simulink model "NN_SMC_Position"  (R2024b)
settings: Solver=ode4  StartTime=0.0  StopTime=200  FixedStep=0.01  RelTol=1e-3
InitFcn:
  |             % distance between camera and world frame
  | ang_initial = [0.0 0.0 0.0];  % initial orientation, [pi 0 pi/2]
  | 
  | init_pose = [C ; ang_initial'];
  | 
  | dT=0.25;
  | g = 9.81;
  | mass = 1; L = 0.2;
  | Ix = 0.008;
  | Iy = 0.008;
  | Iz = 0.017;
  | c = 0.088;
undefined symbols (not defined in the file): C
libraries: ros2lib x2
settings Model: Creator=k513  LastModifiedBy=mohsen
settings DataIOCC: ReturnWorkspaceOutputs=off
settings ModelReferenceCC: EnableRefExpFcnMdlSchedulingChecks=on
settings RTWCC: GPUComputeCapability=3.5

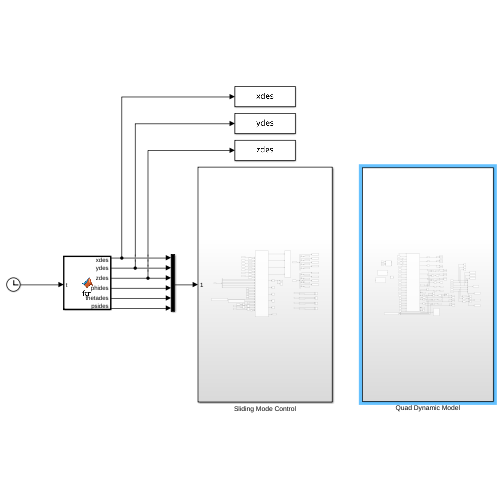
[thumbnail: Simulink's stored preview of the top-level diagram]
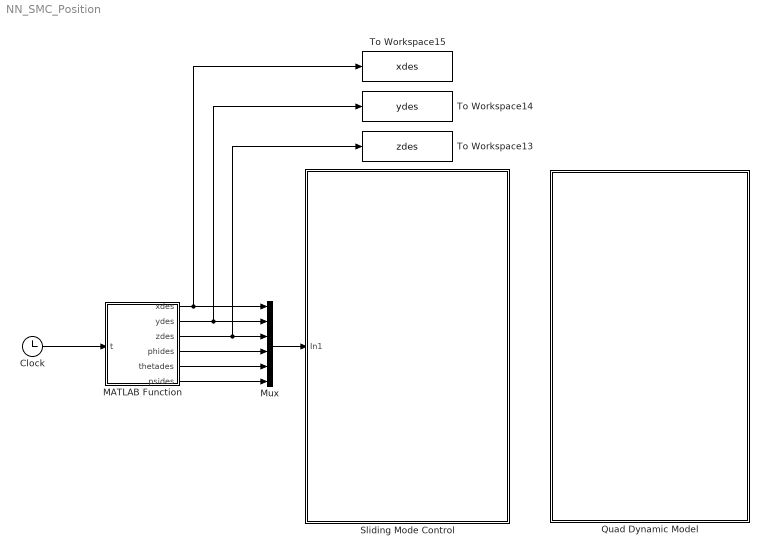
== system NN_SMC_Position ==
  Clock : Clock
  MATLAB Function : MATLAB Function  TreatAsAtomicUnit=on
  Mux : Mux  Inputs=6
  Quad Dynamic Model : Subsystem
  Sliding Mode Control : Subsystem
  To Workspace13 : ToWorkspace  VariableName=zdes  SampleTime=-1
      settings: Save2DSignal=2-D array (concatenate along first dimension)
  To Workspace14 : ToWorkspace  VariableName=ydes  SampleTime=-1
      settings: Save2DSignal=2-D array (concatenate along first dimension)
  To Workspace15 : ToWorkspace  VariableName=xdes  SampleTime=-1
      settings: Save2DSignal=2-D array (concatenate along first dimension)
  wires:
  Clock/1 -> MATLAB Function/1(t)
  Mux/1 -> Sliding Mode Control/1(In1)
  MATLAB Function/1(xdes) -> Mux/1, To Workspace15/1
  MATLAB Function/2(ydes) -> Mux/2, To Workspace14/1
  MATLAB Function/3(zdes) -> Mux/3, To Workspace13/1
  MATLAB Function/4(phides) -> Mux/4
  MATLAB Function/5(thetades) -> Mux/5
  MATLAB Function/6(psides) -> Mux/6

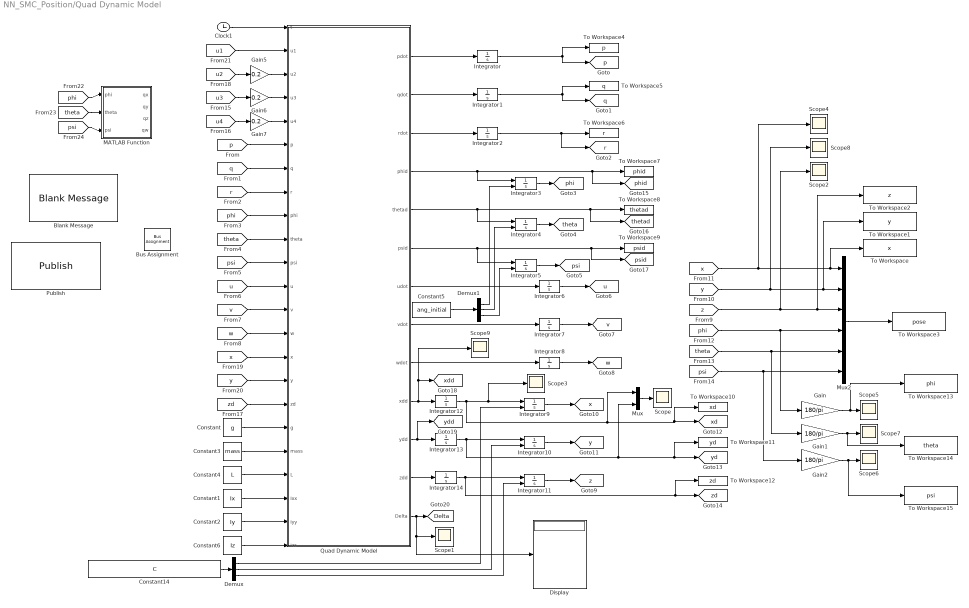
== system NN_SMC_Position/Quad Dynamic Model ==
  Blank Message : ros2lib/Blank Message  messageClass=Message  entityType=geometry_msgs/PoseStamped  messageType=geometry_msgs/PoseStamped  SampleTime=inf
  Bus Assignment : BusAssignment  AssignedSignals=signal1
  Clock1 : Clock
  Constant : Constant  Value=g
  Constant1 : Constant  Value=Ix
  Constant14 : Constant  Value=C
  Constant2 : Constant  Value=Iy
  Constant3 : Constant  Value=mass
  Constant4 : Constant  Value=L
  Constant5 : Constant  Value=ang_initial
  Constant6 : Constant  Value=Iz
  Demux : Demux  Outputs=3
  Demux1 : Demux  Outputs=3
  Display : Display
  Gain : Gain  Gain=180/pi
  Gain1 : Gain  Gain=180/pi
  Gain2 : Gain  Gain=180/pi
  Gain5 : Gain  Gain=0.2
  Gain6 : Gain  Gain=0.2
  Gain7 : Gain  Gain=0.2
  Integrator : Integrator  InitialCondition=-0.003775510005653
  Integrator1 : Integrator  InitialCondition=0.003931066952646
  Integrator{3..5,9..11} (6 alike) : Integrator  InitialConditionSource=external
  Integrator{6..8,12..14} (6 alike) : Integrator
  Integrator2 : Integrator  InitialCondition=0.005723309703171
  MATLAB Function : MATLAB Function  TreatAsAtomicUnit=on
  Mux : Mux  Inputs=2
  Mux2 : Mux  Inputs=6
  Publish : ros2lib/Publish  topicSource=Select from ROS network  topic=/my_topic  messageType=geometry_msgs/Point  QOSHistory=Keep last  QOSDepth=1  QOSReliability=Reliable  QOSDurability=Volatile  QOSDeadline=Inf  QOSLifespan=Inf  QOSLiveliness=Automatic  QOSLeaseDuration=Inf  QOSAvoidROSNamespaceConventions=off
  Quad Dynamic Model : MATLAB Function  TreatAsAtomicUnit=on
  Scope{,1..9} (10 alike) : Scope
  To Workspace : ToWorkspace  VariableName=x  SampleTime=-1
      settings: Save2DSignal=2-D array (concatenate along first dimension)
  To Workspace1 : ToWorkspace  VariableName=y  SampleTime=-1
      settings: Save2DSignal=2-D array (concatenate along first dimension)
  To Workspace10 : ToWorkspace  VariableName=xd  SampleTime=-1
  To Workspace11 : ToWorkspace  VariableName=yd  SampleTime=-1
  To Workspace12 : ToWorkspace  VariableName=zd  SampleTime=-1
  To Workspace13 : ToWorkspace  VariableName=phi  SampleTime=-1
      settings: Save2DSignal=2-D array (concatenate along first dimension)
  To Workspace14 : ToWorkspace  VariableName=theta  SampleTime=-1
      settings: Save2DSignal=2-D array (concatenate along first dimension)
  To Workspace15 : ToWorkspace  VariableName=psi  SampleTime=-1
      settings: Save2DSignal=2-D array (concatenate along first dimension)
  To Workspace2 : ToWorkspace  VariableName=z  SampleTime=-1
      settings: Save2DSignal=2-D array (concatenate along first dimension)
  To Workspace3 : ToWorkspace  VariableName=pose  SampleTime=-1
      settings: Save2DSignal=2-D array (concatenate along first dimension)
  To Workspace4 : ToWorkspace  VariableName=p  SampleTime=-1
  To Workspace5 : ToWorkspace  VariableName=q  SampleTime=-1
  To Workspace6 : ToWorkspace  VariableName=r  SampleTime=-1
  To Workspace7 : ToWorkspace  VariableName=phid  SampleTime=-1
  To Workspace8 : ToWorkspace  VariableName=thetad  SampleTime=-1
  To Workspace9 : ToWorkspace  VariableName=psid  SampleTime=-1
  tag scope: Delta=global, p=global, phi=global, phid=global, psi=global, psid=global, q=global, r=global, theta=global, thetad=global, u=global, v=global, w=global, x=global, xd=global, xdd=global, y=global, yd=global, ydd=global, z=global, zd=global
  wires:
  Quad Dynamic Model/1(pdot) -> Integrator/1
  Quad Dynamic Model/2(qdot) -> Integrator1/1
  Quad Dynamic Model/3(rdot) -> Integrator2/1
  Quad Dynamic Model/4(phid) -> Integrator3/1, [phid], To Workspace7/1
  Quad Dynamic Model/5(thetad) -> Integrator4/1, [thetad], To Workspace8/1
  Quad Dynamic Model/7(udot) -> Integrator6/1
  Quad Dynamic Model/9(wdot) -> Integrator8/1
  Quad Dynamic Model/10(xdd) -> Integrator12/1, Scope9/1, [xdd]
  Quad Dynamic Model/11(ydd) -> Integrator13/1, [ydd]
  Quad Dynamic Model/12(zdd) -> Integrator14/1
  Integrator1/1 -> To Workspace5/1, [q]
  Integrator2/1 -> To Workspace6/1, [r]
  Integrator3/1 -> [phi]
  Integrator4/1 -> [theta]
  Integrator5/1 -> [psi]
  Integrator6/1 -> [u]
  Integrator7/1 -> [v]
  Integrator8/1 -> [w]
  [p] -> Quad Dynamic Model/6(p)
  [q] -> Quad Dynamic Model/7(q)
  [r] -> Quad Dynamic Model/8(r)
  [phi] -> Quad Dynamic Model/9(phi)
  [theta] -> Quad Dynamic Model/10(theta)
  [psi] -> Quad Dynamic Model/11(psi)
  [u] -> Quad Dynamic Model/12(u)
  [v] -> Quad Dynamic Model/13(v)
  [w] -> Quad Dynamic Model/14(w)
  Integrator9/1 -> [x]
  Integrator10/1 -> [y]
  Integrator11/1 -> [z]
  [u2] -> Gain5/1
  [u3] -> Gain6/1
  [u4] -> Gain7/1
  Integrator12/1 -> [xd], To Workspace10/1, Mux/1, Scope3/1, Integrator9/1
  Integrator13/1 -> [yd], To Workspace11/1, Mux/2, Integrator10/1
  Integrator14/1 -> [zd], To Workspace12/1, Integrator11/1
  Quad Dynamic Model/6(psid) -> To Workspace9/1, [psid], Integrator5/1
  Demux/1 -> Integrator9/2
  Demux/2 -> Integrator10/2
  Demux/3 -> Integrator11/2
  Mux/1 -> Scope/1
  Constant14/1 -> Demux/1
  Quad Dynamic Model/8(vdot) -> Integrator7/1
  [x] -> Mux2/1, To Workspace/1, Scope4/1
  [phi] -> Gain/1, Mux2/4
  [psi] -> Mux2/6, Gain2/1
  [theta] -> Gain1/1, Mux2/5
  Gain/1 -> To Workspace13/1, Scope5/1
  Gain1/1 -> Scope7/1, To Workspace14/1
  Gain2/1 -> Scope6/1, To Workspace15/1
  [y] -> Mux2/2, To Workspace1/1, Scope8/1
  [z] -> To Workspace2/1, Mux2/3, Scope2/1
  Mux2/1 -> To Workspace3/1
  Constant/1 -> Quad Dynamic Model/18(g)
  Constant2/1 -> Quad Dynamic Model/22(Iyy)
  Constant1/1 -> Quad Dynamic Model/21(Ixx)
  Constant3/1 -> Quad Dynamic Model/19(mass)
  Constant4/1 -> Quad Dynamic Model/20(L)
  Constant5/1 -> Demux1/1
  Demux1/1 -> Integrator3/2
  Demux1/2 -> Integrator4/2
  Demux1/3 -> Integrator5/2
  Constant6/1 -> Quad Dynamic Model/23(Izz)
  Integrator/1 -> To Workspace4/1, [p]
  [u1] -> Quad Dynamic Model/2(u1)
  Gain5/1 -> Quad Dynamic Model/3(u2)
  Gain6/1 -> Quad Dynamic Model/4(u3)
  Gain7/1 -> Quad Dynamic Model/5(u4)
  [zd] -> Quad Dynamic Model/17(zd)
  Clock1/1 -> Quad Dynamic Model/1(t)
  [x] -> Quad Dynamic Model/15(x)
  [y] -> Quad Dynamic Model/16(y)
  Quad Dynamic Model/13(Delta) -> Display/1, Scope1/1, [Delta]
  [phi] -> MATLAB Function/1(phi)
  [theta] -> MATLAB Function/2(theta)
  [psi] -> MATLAB Function/3(psi)

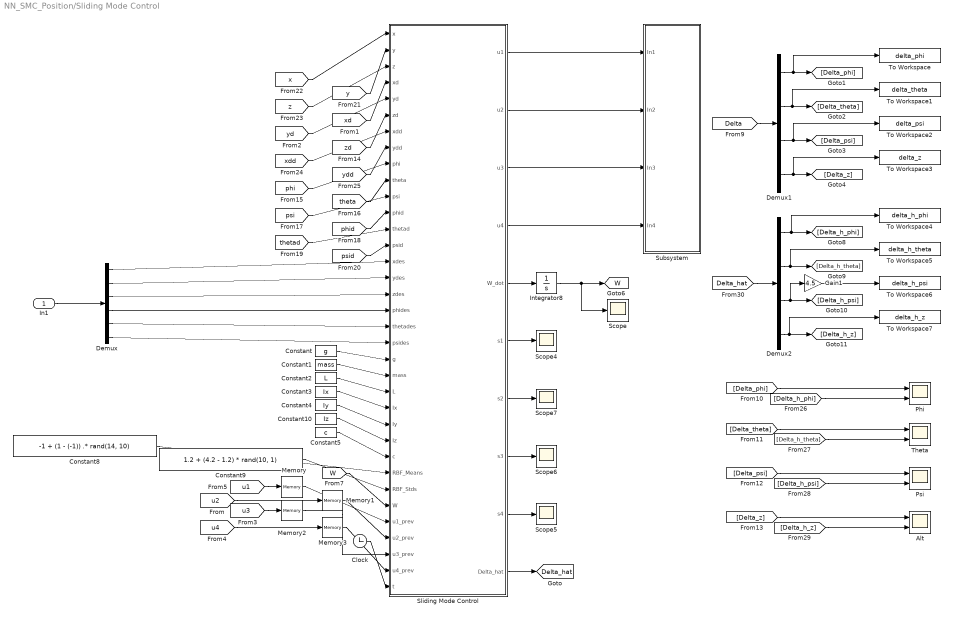
== system NN_SMC_Position/Sliding Mode Control ==
  In1 : Inport
  Alt : Scope  NumInputPorts=2
  Clock : Clock
  Constant : Constant  Value=g
  Constant1 : Constant  Value=mass
  Constant10 : Constant  Value=Iz
  Constant2 : Constant  Value=L
  Constant3 : Constant  Value=Ix
  Constant4 : Constant  Value=Iy
  Constant5 : Constant  Value=c
  Constant8 : Constant  Value=-1 + (1 - (-1)) .* rand(14, 10)
  Constant9 : Constant  Value=1.2 + (4.2 - 1.2) * rand(10, 1)
  Demux : Demux  Outputs=6
  Demux1 : Demux
  Demux2 : Demux
  Gain1 : Gain  Gain=4.5
  Integrator8 : Integrator  InitialCondition=zeros(10, 4)
  Memory{,1..3} (4 alike) : Memory
  Phi : Scope  NumInputPorts=2
  Psi : Scope  NumInputPorts=2
  Scope{,4..7} (5 alike) : Scope
  Sliding Mode Control : MATLAB Function  TreatAsAtomicUnit=on
  Subsystem : Subsystem
  Theta : Scope  NumInputPorts=2
  To Workspace : ToWorkspace  VariableName=delta_phi  SampleTime=-1
      settings: Save2DSignal=2-D array (concatenate along first dimension)
  To Workspace1 : ToWorkspace  VariableName=delta_theta  SampleTime=-1
      settings: Save2DSignal=2-D array (concatenate along first dimension)
  To Workspace2 : ToWorkspace  VariableName=delta_psi  SampleTime=-1
      settings: Save2DSignal=2-D array (concatenate along first dimension)
  To Workspace3 : ToWorkspace  VariableName=delta_z  SampleTime=-1
      settings: Save2DSignal=2-D array (concatenate along first dimension)
  To Workspace4 : ToWorkspace  VariableName=delta_h_phi  SampleTime=-1
      settings: Save2DSignal=2-D array (concatenate along first dimension)
  To Workspace5 : ToWorkspace  VariableName=delta_h_theta  SampleTime=-1
      settings: Save2DSignal=2-D array (concatenate along first dimension)
  To Workspace6 : ToWorkspace  VariableName=delta_h_psi  SampleTime=-1
      settings: Save2DSignal=2-D array (concatenate along first dimension)
  To Workspace7 : ToWorkspace  VariableName=delta_h_z  SampleTime=-1
      settings: Save2DSignal=2-D array (concatenate along first dimension)
  tag scope: Delta_hat=global, W=global
  wires:
  [theta] -> Sliding Mode Control/10(theta)
  [zd] -> Sliding Mode Control/6(zd)
  [yd] -> Sliding Mode Control/5(yd)
  [xdd] -> Sliding Mode Control/7(xdd)
  [thetad] -> Sliding Mode Control/13(thetad)
  [phid] -> Sliding Mode Control/12(phid)
  [psi] -> Sliding Mode Control/11(psi)
  [ydd] -> Sliding Mode Control/8(ydd)
  [y] -> Sliding Mode Control/2(y)
  [phi] -> Sliding Mode Control/9(phi)
  [xd] -> Sliding Mode Control/4(xd)
  [psid] -> Sliding Mode Control/14(psid)
  [x] -> Sliding Mode Control/1(x)
  [z] -> Sliding Mode Control/3(z)
  In1/1 -> Demux/1
  Demux/1 -> Sliding Mode Control/15(xdes)
  Demux/2 -> Sliding Mode Control/16(ydes)
  Demux/3 -> Sliding Mode Control/17(zdes)
  Constant/1 -> Sliding Mode Control/21(g)
  Constant1/1 -> Sliding Mode Control/22(mass)
  Constant2/1 -> Sliding Mode Control/23(L)
  Constant3/1 -> Sliding Mode Control/24(Ix)
  Constant4/1 -> Sliding Mode Control/25(Iy)
  Constant5/1 -> Sliding Mode Control/27(c)
  Demux/5 -> Sliding Mode Control/19(thetades)
  Demux/6 -> Sliding Mode Control/20(psides)
  Demux/4 -> Sliding Mode Control/18(phides)
  Constant10/1 -> Sliding Mode Control/26(Iz)
  Constant9/1 -> Sliding Mode Control/29(RBF_Stds)
  Constant8/1 -> Sliding Mode Control/28(RBF_Means)
  Sliding Mode Control/5(W_dot) -> Integrator8/1
  [u1] -> Memory/1
  [u2] -> Memory1/1
  [u3] -> Memory2/1
  [u4] -> Memory3/1
  Sliding Mode Control/6(s1) -> Scope4/1
  Sliding Mode Control/9(s4) -> Scope5/1
  Sliding Mode Control/8(s3) -> Scope6/1
  Sliding Mode Control/7(s2) -> Scope7/1
  Memory/1 -> Sliding Mode Control/31(u1_prev)
  Memory1/1 -> Sliding Mode Control/32(u2_prev)
  Memory2/1 -> Sliding Mode Control/33(u3_prev)
  Memory3/1 -> Sliding Mode Control/34(u4_prev)
  Sliding Mode Control/10(Delta_hat) -> [Delta_hat]
  Integrator8/1 -> Scope/1, [W]
  [W] -> Sliding Mode Control/30(W)
  Sliding Mode Control/1(u1) -> Subsystem/1(In1)
  Sliding Mode Control/2(u2) -> Subsystem/2(In2)
  Sliding Mode Control/3(u3) -> Subsystem/3(In3)
  Sliding Mode Control/4(u4) -> Subsystem/4(In4)
  Clock/1 -> Sliding Mode Control/35(t)
  [Delta_phi] -> Phi/1
  Demux1/2 -> To Workspace1/1, [Delta_theta]
  [Delta_h_theta] -> Theta/2
  Gain1/1 -> To Workspace6/1
  Demux1/1 -> To Workspace/1, [Delta_phi]
  Demux1/4 -> To Workspace3/1, [Delta_z]
  Demux2/4 -> To Workspace7/1, [Delta_h_z]
  Demux2/1 -> To Workspace4/1, [Delta_h_phi]
  [Delta_theta] -> Theta/1
  [Delta_h_psi] -> Psi/2
  Demux1/3 -> To Workspace2/1, [Delta_psi]
  Demux2/3 -> Gain1/1, [Delta_h_psi]
  [Delta_h_z] -> Alt/2
  [Delta] -> Demux1/1
  [Delta_hat] -> Demux2/1
  [Delta_psi] -> Psi/1
  [Delta_h_phi] -> Phi/2
  Demux2/2 -> To Workspace5/1, [Delta_h_theta]
  [Delta_z] -> Alt/1

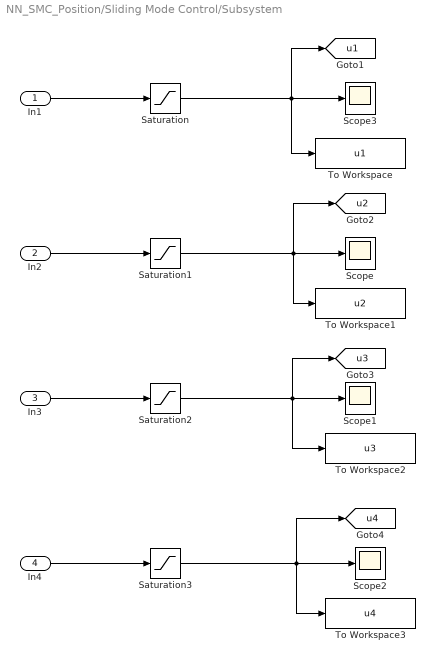
== system NN_SMC_Position/Sliding Mode Control/Subsystem ==
  In1 : Inport
  In2 : Inport  Port=2
  In3 : Inport  Port=3
  In4 : Inport  Port=4
  Saturation : Saturate  UpperLimit=400  LowerLimit=-350
  Saturation1 : Saturate  UpperLimit=8  LowerLimit=-8
  Saturation2 : Saturate  UpperLimit=8  LowerLimit=-8
  Saturation3 : Saturate  UpperLimit=4  LowerLimit=-3
  Scope{,1..3} (4 alike) : Scope
  To Workspace : ToWorkspace  VariableName=u1  SaveFormat=Timeseries  SampleTime=-1
  To Workspace1 : ToWorkspace  VariableName=u2  SaveFormat=Timeseries  SampleTime=-1
  To Workspace2 : ToWorkspace  VariableName=u3  SaveFormat=Timeseries  SampleTime=-1
  To Workspace3 : ToWorkspace  VariableName=u4  SaveFormat=Timeseries  SampleTime=-1
  tag scope: u1=global, u2=global, u3=global, u4=global
  wires:
  Saturation/1 -> Scope3/1, To Workspace/1, [u1]
  In4/1 -> Saturation3/1
  Saturation2/1 -> [u3], Scope1/1, To Workspace2/1
  In3/1 -> Saturation2/1
  Saturation3/1 -> [u4], Scope2/1, To Workspace3/1
  In2/1 -> Saturation1/1
  Saturation1/1 -> To Workspace1/1, Scope/1, [u2]
  In1/1 -> Saturation/1

== matlab function NN_SMC_Position/Quad Dynamic Model/MATLAB Function ==
  data: phi input; qx output; theta input; psi input; qy output; qz output; qw output
function [qx,qy,qz,qw] = eul2quat_simu(phi,theta,psi)

cy = cos(psi*0.5);
sy = sin(psi*0.5);
cp = cos(theta*0.5);
sp = sin(theta*0.5);
cr = cos(phi*0.5);
sr = sin(phi*0.5);

qw = cr*cp*cy + sr*sp*sy;
qx = sr*cp*cy - cr*sp*sy;
qy = cr*sp*cy + sr*cp*sy;
qz = cr*cp*sy - sr*sp*cy;

== matlab function NN_SMC_Position/Sliding Mode Control/Sliding Mode Control ==
  data: u1 output; x input; y input; z input; xd input; yd input; zd input; xdd input; ydd input; phi input; theta input; psi input; phid input; thetad input; psid input; xdes input; ydes input; zdes input; phides input; thetades input; u2 output; u3 output; u4 output; psides input; g input; mass input; L input; Ix input; Iy input; Iz input; c input; RBF_Means input; RBF_Stds input; W_dot output; W input; u1_prev input; u2_prev input; u3_prev input; u4_prev input; s1 output; s2 output; s3 output; s4 output; Delta_hat output; t input
function [u1, u2, u3, u4, W_dot, s1,s2,s3,s4, Delta_hat]     = fcn(x,y,z,xd,yd,zd,xdd,ydd,phi,theta,psi,phid,thetad,psid, xdes, ydes, zdes,phides, thetades,psides,g,mass,L,Ix,Iy,Iz, c, RBF_Means, RBF_Stds, W, u1_prev, u2_prev, u3_prev, u4_prev, t)

phiddes = 0;
phidddes = 0;
thetaddes = 0;
thetadddes = 0;
xddes = 0;
xdddes = 0;
yddes = 0;
ydddes = 0;
zddes = 0;
zdddes = 0;
psiddes = 0;
psidddes = 0;
%if zdes<0
%zdes=0.5;
%end

%% NN
% neural net inputs
Gamma = 200;
e_dot_z = zd - zddes;
x_n = [phi/10; theta/10; 50*psi/1; z/10; zdes/15];
x_dot_n = [phid/10; thetad/10; 50*psid/1; zd/10; e_dot_z*2];
u = [u2_prev; u3_prev; u4_prev; u1_prev];
u_n = u/15;
nn_input = [x_n; x_dot_n; u_n];


mu = zeros(10, 1);
for i = 1 : 10
    mu(i, 1) = exp(-norm(nn_input - RBF_Means(:, i))^2/(2 * RBF_Stds(i)^2));
end

% estimation of uncertainties
Delta_hat = transpose(W) * mu;


%%
ghat = 1 * g; cz = 1; masshat = mass;
eps1 = 0.8;
eta1 = 20;
s1 = cz*(z - zdes) + (zd - zddes);
s1 = tanh(s1);
u1 = (masshat/(cos(phi)*cos(theta)))*(cz*(zd-zddes) - zdddes + ghat + eta1*s1 + Delta_hat(4));
%%%%%%%%%%%%%%%%%%%%%%%%%%%%%%%
% if s1 > 1
%     sgn1 = 1;
% elseif   s1 < -1
%     sgn1 = -1;
% else
%     sgn1 = s1;
% end
% u1 = (masshat/(cos(phi)*cos(theta)))*(cz*(zd-zddes) - zdddes + ghat + eps1*sgn1 + eta1*s1 + Delta_hat(4));
%%%%%%%%%%%%%%%%%%%%%%%%%%%%%%%

%%
cpsi = 1.5; eps2 = 0.8; eta2 = 10; 
Izhat = 1 * Iz; chat = 1 * c;
s2 = +cpsi*(psi - psides) + (psid - psiddes);
s2 = tanh(s2);
u4 = (Izhat/chat)*(-(Ix-Iy/Iz)*phid*thetad - cpsi*(psid-psiddes) + psidddes - eta2*s2 + 0.43*Delta_hat(3));
% if s2 > 1
%     sgn2 = 1;
% elseif   s2 < -1
%     sgn2 = -1;
% else
%     sgn2 = s2;
% end
% u4 = (Izhat/chat)*(cpsi*(psiddes-psid) + psidddes + eps2*sgn2 + eta2*s2 + 2*Delta_hat(3));
%% 
eps3 = 0.5; eta3 = 50; ctheta = 1.5;
Iyhat = 1 * Iy; Ixhat = 1 * Ix; lhat = 1 * L;
c3 = 1;
c1 = (11*mass/(u1*cos(phi)*cos(psi)*cos(thetades))) * c3;
c2 = (6*mass/(u1*cos(phi)*cos(psi)*cos(thetades))) * c3;
% c1 = (11*mass/(cos(phi)*cos(psi)*cos(thetades))) * c3;
% c2 = (6*mass/(cos(phi)*cos(psi)*cos(thetades))) * c3;
c4 = (6) * c3;
s3 = c1*(xddes - xd) + c2*(xdes - x) + c3*(thetaddes - thetad) + c4*(thetades - theta);

% s3 = c3*(thetaddes - thetad) + c4*(thetades- theta);

% if s3 > 1
%     sgn3 = 1;
% elseif   s3 < -1
%     sgn3 = -1;
% else
%     sgn3 = s3;
% end
s3 = tanh(s3);
u3 = (Iyhat/lhat)*((c1/c3)*(xdddes-xdd) + (c2/c3)*(xddes-xd) + thetadddes ...
       + (c4/c3)*(thetaddes-thetad)  + (1/c3)*(eta3*s3) + Delta_hat(2));

% u3 = (Iyhat/lhat)*((c1/c3)*(xdddes-xdd) + (c2/c3)*(xddes-xd) + thetadddes ...
%        + (c4/c3)*(thetaddes-thetad)  + (1/c3)*(eps3*sgn3 + eta3*s3) + Delta_hat(2));
% u3 = (Iyhat/chat)*(ctheta*(thetaddes-thetad) + thetadddes + eps3*sgn3 + eta3*s3);

%u3(st) = 0;
%%
eps4 = 0.5; eta4 = 50; chphi = 1.5;
c7 = 1;
% c5 = (-11*mass/((u1*sin(phides)*sin(theta)*sin(psi))+(u1*cos(phides)*cos(psi)))) * c7;
% c6 = (-6*mass/((u1*sin(phides)*sin(theta)*sin(psi))+(u1*cos(phides)*cos(psi)))) * c7;
% c5 = (-11*mass/((sin(phides)*sin(theta)*sin(psi))+(u1*cos(phides)*cos(psi)))) * c7;
% c6 = (-6*mass/((sin(phides)*sin(theta)*sin(psi))+(u1*cos(phides)*cos(psi)))) * c7;
c5 = (-11*mass/((sin(phides)*sin(theta)*sin(psi))+(cos(phides)*cos(psi)))) * c7;
c6 = (-6*mass/((sin(phides)*sin(theta)*sin(psi))+(cos(phides)*cos(psi)))) * c7;
c8 = (6) * c7;

s4 = c5*(yddes - yd) + c6*(ydes - y) + c7*(phiddes - phid) + c8*(phides - phi);

% s4 = c7*(phiddes - phid) + c8*(phides - phi);
if s4 > 1
    sgn4 = 1;
elseif   s4 < -1
    sgn4 = -1;
else
    sgn4 = s4;
end
u2 = (Ixhat/lhat)*((c5/c7)*(ydddes-ydd) + (c6/c7)*(yddes-yd) + phidddes ...
        + (c8/c7)*(phiddes-phid) +  (1/c7)*(eps4*sgn4 + eta4*s4) + Delta_hat(1));
% u2 = (Ixhat/lhat)*(chphi*(phiddes-phid) + phidddes + eps4*sgn4 + eta4*s4);

s = [s4; s3; -s2; 2*s1];
% s = s3_nn;
W_dot = Gamma * mu * s';


%);%

== matlab function NN_SMC_Position/MATLAB Function ==
  data: t input; xdes output; ydes output; zdes output; phides output; thetades output; psides output
function [xdes, ydes, zdes, phides, thetades, psides] = fcn(t)
%FCN defines a piecewise square-like reference trajectory over 50s

% Desired angles (all zero)
phides   = 0;
thetades = 0;
psides   = 0;

% Desired altitude (linear)
zdes = 2;



if t < 15
    xdes = 0;
    ydes = t / 15;              % y: 0 → 1
elseif t < 30
    xdes = (t - 15) / 15;       % x: 0 → 1
    ydes = 1;
elseif t < 45
    xdes = 1;
    ydes = 1 - (t - 30) / 15;   % y: 1 → 0
elseif t <= 60
    xdes = 1 - (t - 45) / 15;   % x: 1 → 0
    ydes = 0;
else
    xdes = 0;
    ydes = 0;
    zdes = 0;
end

end

== matlab function NN_SMC_Position/Quad Dynamic Model/Quad Dynamic Model ==
  data: t input; u1 input; u2 input; u3 input; u4 input; p input; pdot output; q input; r input; qdot output; rdot output; phi input; theta input; psi input; u input; v input; w input; x input; y input; zd input; phid output; thetad output; psid output; udot output; vdot output; wdot output; xdd output; ydd output; zdd output; g input; mass input; L input; Ixx input; Iyy input; Izz input; Delta output
function [pdot, qdot, rdot, phid, thetad, psid, udot, vdot, wdot, xdd, ydd, zdd, Delta] = fcn(t, u1, u2, u3, u4, p, q, r, phi, theta, psi, u, v, w, x, y, zd, g, mass, L, Ixx, Iyy, Izz)


% k1 = 0.1; k2 = 0.1; k3 = 0.1; k4 = 0.12; k5 = 0.12; k6 = 0.12;
 
%Izz = Ixx+Iyy;

phid = p + q*sin(phi)*tan(theta) + r*cos(phi)*tan(theta);
thetad = q*cos(phi) - r*sin(phi);
psid = q*sin(phi)*sec(theta) + r*cos(phi)*sec(theta);

Delta1 = [phi * theta; theta * psi; phi * psi; 0.2 * zd];
d1 = [10*0.5 * sin(pi * t/2); 10*0.5 * sin(pi * t/3); 10*0.2 * sin(pi * t); 6*sin(2 * pi * t + pi/6)];
Delta = Delta1 + d1;

pdot = r*q*(Iyy - Izz)/Ixx + (u2)/Ixx - Delta(1);
qdot = r*p*(Izz - Ixx)/Iyy + (u3)/Iyy - Delta(2);
rdot = p*q*(Ixx - Iyy)/Izz + (u4)/Izz - Delta(3);


udot = r*v - q*w -g*sin(theta);
vdot = p*w - u*r +g*cos(theta)*sin(phi); 
wdot = q*u - p*v +g*cos(theta)*cos(phi) - u1/mass;

% AA = [cos(psi)*cos(theta), -sin(psi)*cos(phi)+cos(psi)*sin(theta)*sin(phi), sin(psi)*sin(phi)+cos(psi)*sin(theta)*cos(phi);
%      sin(psi)*cos(theta), cos(psi)*cos(phi)+sin(psi)*sin(theta)*sin(phi), -sin(phi)*cos(psi)+sin(psi)*sin(theta)*cos(phi);
%     -sin(theta), cos(theta)*sin(phi), cos(theta)*cos(phi)]; 
% 
% xd = AA(1,:)*[u;v;w];
% yd = AA(2,:)*[u;v;w];
% zd = AA(3,:)*[u;v;w];

% xdd = (-u1/mass)*(sin(phi)*sin(psi)+cos(phi)*cos(psi)*sin(theta));
% ydd = (-u1/mass)*(cos(phi)*sin(psi)*sin(theta)-cos(psi)*sin(phi));
% zdd = g + (-u1/mass)*(cos(phi)*cos(theta));

xdd = (1/mass)*(cos(phi)*sin(theta)*cos(psi)+sin(phi)*sin(psi))*u1 ;
ydd = (1/mass)*(sin(psi)*sin(theta)*cos(phi)-cos(psi)*sin(phi))*u1 ;
zdd = -(1/mass)*(cos(phi)*cos(theta))*u1+g + Delta(4);
